simulink model "Discharging"  (R2021a)
settings: Solver=VariableStepAuto  StartTime=0.0  StopTime=6000  RelTol=1e-3
undefined symbols (not defined in the file or in its folder): Ion, Lithium
libraries: spsStairGeneratorLib x1, spsBatteryLib x1, spsCurrentMeasurementLib x1, spsMosfetLib x1, spsSeriesRLCBranchLib x1, spsVoltageMeasurementLib x1, spspowerguiLib x1
settings Model: Creator=Samiran  LastModifiedBy=Samiran

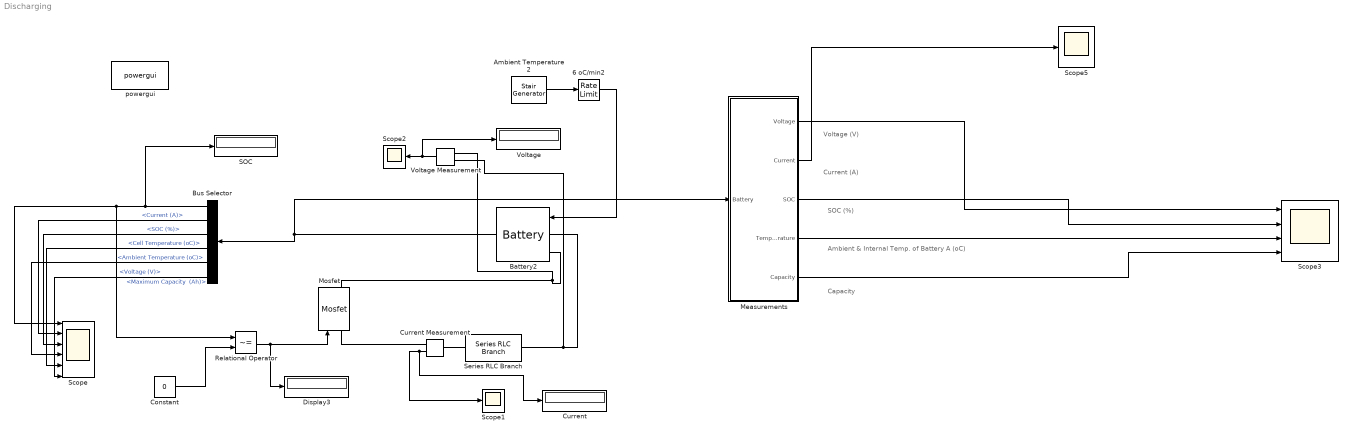
== system Discharging ==
  note: Capacity
  note: SOC (%)
  note: Ambient & Internal Temp. of Battery A (oC)
  note: Current (A)
  note: Voltage (V)
  6 oC/min2 : RateLimiter  RisingSlewLimit=0.5  FallingSlewLimit=-0.5  SampleTimeMode=inherited
  Ambient Temperature2 : spsStairGeneratorLib/Stair Generator  t="[0, 500, 1000 1500  2000 2500 3000]"  e="[20, 0, -20  0  20, 50 20]"  Ts=0
  Battery2 : spsBatteryLib/Battery  BatType=Lithium-Ion  ShowTempParam=on  ThermalPreset="3.6V  3.6Ah  (LiNiO2)"  ShowAgeParam=on  NomV=3.1  NomQ=3.6  SOC=96  Batt_Tr=30  PresetModel=off  MaxQ=3.2  MinV=2.325  FullV=3.75  Dis_rate=0.72  R=0.00889  Normal_OP=2.8  expZone="[3.5         0.5]"  current=[6.5 13 32.5]  Units=Time  Tci=20  NomT=20  T2=0  MaxQ2=2.7  FullV2=3.5  Normal_OP2=2.94  expZone2="[3.25         0.5]"  Rca=0.6  ti=1000  Dp=0  Neq0=0  Tsim=1e6  Ta1=25  Qeol=5.4*0.9  Reol=0.013333*1.2  Char_age=[2.3478, 3]  Dis_age=[2.3478, 10]  N1=1500  N2=10500  N3=1000  N4=1400  Ta2=45  N5=950
  Bus Selector : BusSelector  OutputSignals="Voltage (V),Current (A),SOC (%),Cell Temperature (oC),Ambient Temperature (oC),Maximum Capacity  (Ah)"
  Constant : Constant  Value=0
  Current : Display
  Current Measurement : spsCurrentMeasurementLib/Current Measurement  PhasorSimulation=off  OutputType=Complex  PSBequivalent=0
  Display3 : Display
  Measurements : Subsystem
  Mosfet : spsMosfetLib/Mosfet  Ron=0.1  Lon=0  Rd=0.01  Vfd=0  IC=0  Rs=1e5  Cs=inf  Measurements=on
  Relational Operator : RelationalOperator  Operator=~=  OutDataTypeStr=boolean  RndMeth=Simplest
  SOC : Display
  Scope : Scope  NumInputPorts=6
  Scope1 : Scope
  Scope2 : Scope
  Scope3 : Scope  NumInputPorts=4
  Scope5 : Scope
  Series RLC Branch : spsSeriesRLCBranchLib/Series RLC Branch  LConnTagsString=__new0  RConnTagsString=__new0  BranchType=R  Resistance=4.4  Inductance=1e-3  SetiL0=off  InitialCurrent=0  Capacitance=1e-6  Setx0=off  InitialVoltage=0  Measurements=None
  Voltage : Display
  Voltage Measurement : spsVoltageMeasurementLib/Voltage Measurement  PhasorSimulation=off  OutputType=Complex  PSBequivalent=0
  powergui : spspowerguiLib/powergui  Priority=1  SimulationMode=Continuous  SampleTime=50e-6  frequency=60  Iterations=50  frequencyindice=0  Pbase=100e6  ErrMax=1e-4  UnitsV=kV  UnitsW=MW  buscounter=0  FunctionMessages=off  echomessages=off  EnableUseOfTLC=off  CurrentSourceSwitches=off  DisableSnubberDevices=off  DisableRonSwitches=off  DisableVfSwitches=off  DisplayEquations=off  AutomaticDiscreteSolvers=off  SolverType=Tustin/Backward Euler (TBE)  Interpol=off  ExternalGateDelay=off  methode=off  Ts=100  x0status=blocks  SPID=on  SwTol=0  HookPort=off  NonlinearTolerance=1e-4  nMaxIteration=100  ContinueOnMaxIteration=off  RestoreLinks=warning  ResistiveCurrentMeasurement=off  Frange=[0:2:500]  Ylog=off  Xlog=on  ShowGrid=off  save=off  variable=ZData  structure=0  ZoomFFT=off  StartTime=0.0  cycles=1  DisplayStyle=1  fundamental=60  FreqAxis=off  MaxFrequency=1000  frequencyindicesteady=1  RmsSteady=1  display=off
  wires:
  Measurements/3(SOC) -> Scope3/2
  Battery2/1 -> Bus Selector/1, Measurements/1("Battery ")
  Voltage Measurement/1 -> Voltage/1, Scope2/1
  Current Measurement/1 -> Current/1, Scope1/1
  Relational Operator/1 -> Display3/1, Mosfet/1
  Constant/1 -> Relational Operator/2
  Bus Selector/1 -> Relational Operator/1, Scope/1, SOC/1  "<Voltage (V)>"
  Ambient Temperature2/1 -> 6 oC/min2/1
  6 oC/min2/1 -> Battery2/1
  Measurements/4(Temperature) -> Scope3/3
  Measurements/5(Capacity) -> Scope3/4
  Bus Selector/2 -> Scope/2  "<Current (A)>"
  Bus Selector/3 -> Scope/3  "<SOC (%)>"
  Bus Selector/4 -> Scope/5  "<Cell Temperature (oC)>"
  Bus Selector/6 -> Scope/6  "<Maximum Capacity  (Ah)>"
  Measurements/2(Current) -> Scope5/1
  Measurements/1(Voltage) -> Scope3/1
  Bus Selector/5 -> Scope/4  "<Ambient Temperature (oC)>"
  connections:
  Series RLC Branch/RConn1 -- Battery2/LConn1 -- Voltage Measurement/LConn1
  Current Measurement/LConn1 -- Series RLC Branch/LConn1
  Mosfet/LConn1 -- Current Measurement/RConn1
  Voltage Measurement/LConn2 -- Battery2/LConn2 -- Mosfet/RConn1

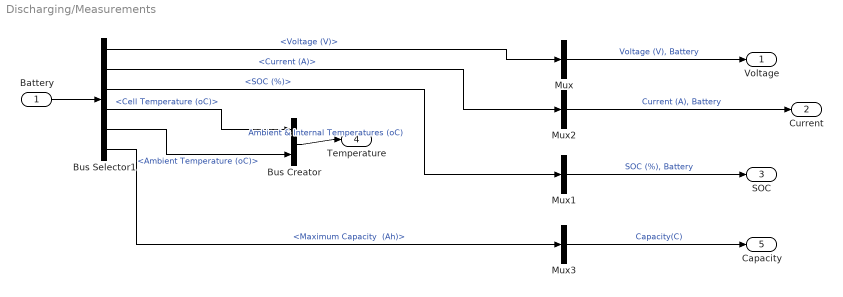
== system Discharging/Measurements ==
  "Battery " : Inport
  Bus Creator : BusCreator  Inputs=2
  Bus Selector1 : BusSelector  OutputSignals="Voltage (V),Current (A),SOC (%),Cell Temperature (oC),Ambient Temperature (oC),Maximum Capacity  (Ah)"
  Mux{,1..3} (4 alike) : Mux  Inputs=1
  Voltage : Outport  VectorParamsAs1DForOutWhenUnconnected=off
  Current : Outport  Port=2  VectorParamsAs1DForOutWhenUnconnected=off
  SOC : Outport  Port=3  VectorParamsAs1DForOutWhenUnconnected=off
  Temperature : Outport  Port=4  VectorParamsAs1DForOutWhenUnconnected=off
  Capacity : Outport  Port=5  VectorParamsAs1DForOutWhenUnconnected=off
  wires:
  Bus Selector1/4 -> Bus Creator/1  "<Cell Temperature (oC)>"
  Bus Selector1/5 -> Bus Creator/2  "<Ambient Temperature (oC)>"
  Bus Creator/1 -> Temperature/1  "Ambient & Internal Temperatures (oC)"
  Bus Selector1/3 -> Mux1/1  "<SOC (%)>"
  Mux1/1 -> SOC/1  "SOC (%), Battery"
  Mux/1 -> Voltage/1  "Voltage (V), Battery"
  Bus Selector1/1 -> Mux/1  "<Voltage (V)>"
  Bus Selector1/2 -> Mux2/1  "<Current (A)>"
  Mux2/1 -> Current/1  "Current (A), Battery"
  "Battery "/1 -> Bus Selector1/1
  Bus Selector1/6 -> Mux3/1  "<Maximum Capacity  (Ah)>"
  Mux3/1 -> Capacity/1  "Capacity(C)"
